simulink model "ACC"  (R2018b)
settings: Solver=ode45  StartTime=0.0  StopTime=80.0  MaxStep=1e-2  RelTol=1e-3
values from neighbouring files (symbols this model uses):
  a = 200    [ACC_param.m]    (also in CriticalVelocity.m = 1.5)
  b = 10000    [ACC_param.m]    (also in CriticalVelocity.m = 1.3)
  kd = (a - 3*p*m)/b    (= -0.082)    [ACC_param.m]
  ki = -(p^3*m)/b    (= -0.0039304)    [ACC_param.m]
  kp = -(3*p^2*m)/b    (= -0.03468)    [ACC_param.m]
  m = 1000    [ACC_param.m]    (also in CriticalVelocity.m = 1700)
settings Model: Creator=jofr  LastModifiedBy=barka
settings DataIOCC: LimitDataPoints=on  SaveFormat=Array  SignalLoggingSaveFormat=ModelDataLogs
settings OptimizationCC: BlockReduction=off  BooleanDataType=off  LifeSpan=inf
settings DebuggingCC: SaveWithParameterizedLinksMsg=none  UnderspecifiedInitializationDetection=Classic  MergeDetectMultiDrivingBlocksExec=none  SignalResolutionControl=TryResolveAllWithWarning  MultiTaskDSMMsg=warning  MultiTaskCondExecSysMsg=none  SFUnexpectedBacktrackingDiag=warning  SFNoUnconditionalDefaultTransitionDiag=warning  SFExecutionAtInitializationDiag=none
settings HardwareCC: ProdBitPerPointer=32  ProdBitPerSizeT=32  ProdBitPerPtrDiffT=32  ProdLargestAtomicFloat=None  ProdIntDivRoundTo=Undefined  ProdEndianess=Unspecified  ProdWordSize=32  ProdHWDeviceType=32-bit Generic  TargetUnknown=on
settings ModelReferenceCC: PropagateSignalLabelsOutOfModel=off
settings SFSimCC: SimUseLocalCustomCode=off
settings RTWCC: RTWUseLocalCustomCode=off
settings CodeAppCC: StateflowObjectComments=on
settings GRTTargetCC: TargetLangStandard=C89/C90 (ANSI)  GeneratePreprocessorConditionals=Disable all
settings ConfigComp: CovMetricSettings=dw  CovHtmlReporting=on  CovSaveCumulativeToWorkspaceVar=on  CovSaveSingleToWorkspaceVar=on  CovExternalEMLEnable=off

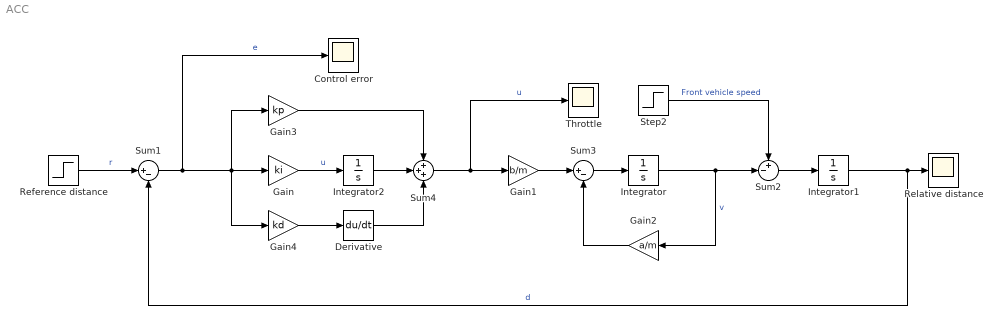
== system ACC ==
  Control error : Scope
  Derivative : Derivative
  Gain : Gain  Gain=ki
  Gain1 : Gain  Gain=b/m
  Gain2 : Gain  Gain=a/m
  Gain3 : Gain  Gain=kp
  Gain4 : Gain  Gain=kd
  Integrator : Integrator  InitialCondition=25
  Integrator1 : Integrator  InitialCondition=25
  Integrator2 : Integrator  InitialCondition=0.5
  Reference distance : Step  Time=0  Before=25  After=25  SampleTime=0
  Relative distance : Scope
  Step2 : Step  Time=20  Before=25  After=13.889  SampleTime=0
  Sum1 : Sum  Inputs=|+-
  Sum2 : Sum  Inputs=+-|
  Sum3 : Sum  Inputs=|+-
  Sum4 : Sum  Inputs=+++
  Throttle : Scope
  wires:
  Sum3/1 -> Integrator/1
  Integrator/1 -> Sum2/2, Gain2/1  "v"
  Sum1/1 -> Control error/1, Gain3/1, Gain4/1, Gain/1  "e"
  Reference distance/1 -> Sum1/1  "r"
  Gain1/1 -> Sum3/1
  Gain2/1 -> Sum3/2
  Integrator1/1 -> Sum1/2, Relative distance/1  "d"
  Sum2/1 -> Integrator1/1
  Step2/1 -> Sum2/1  "Front vehicle speed"
  Sum4/1 -> Throttle/1, Gain1/1  "u"
  Gain3/1 -> Sum4/1
  Gain/1 -> Integrator2/1  "u"
  Gain4/1 -> Derivative/1
  Integrator2/1 -> Sum4/2
  Derivative/1 -> Sum4/3
